simulink library "engine_AMT280_lib"  (Simulink 6.6)
libraries: simulink x5
settings Model: Creator=amurch  LastModifiedBy=amurch

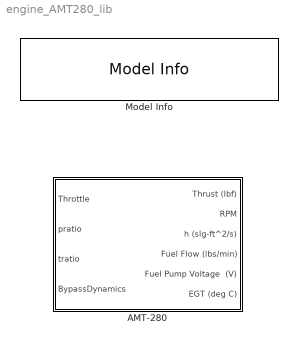
== system engine_AMT280_lib ==
  AMT-280 : Subsystem
      mask init:
      | % Curve fit parameters for AMT-280 Model
      | Coeff_thrust   = [ 5.7372e-05  -5.2629e-03   3.1586e-01  -5.1517e+00];
      | Coeff_throttle = [ -4.3078e-03   1.1110e+00   2.9012e+01];
      | Coeff_fuelflow = [ 1.0140e-04  -1.5867e-03   2.0125e-01];
      | Coeff_tau      = [ -2.2400e-02   2.9948e+00];
      | 
      | 
      | % Equvalent Shaft parameters for engine
      | shaft_dia = 0.75/12.0;       % diameter of rotating turbine in feet 
      | shaft_len = 6.25/12.0;       % length of rotating turbine in feet   
      | density   = 15.2;            % mass density of steel in slugs/ft^3 
      | 
      | fuelpump_table = [ 0.90 1.0 6.4]; %volts, table of fuel pump voltages  - not accurate at the moment 2-4-08
      | fuelflow_table = [0.00 0.1762 1.34044]; %lbs/min,   fuel flow rates corresponding to pump voltages (pumpv_table)
  Model Info : simulink/Model-Wide Utilities/Model Info  SystemSampleTime=-1  InitialBlockCM=None  BlockCM=None  Frame=on  DisplayStringWithTags=|  HorizontalTextAlignment=Center  LeftAlignmentValue=0.5  SourceBlockDiagram=engine_AMT280_lib  TagMaxNumber=20
      | AMT-280 Engine Library
      | 
      | Model Version: %<ModelVersion>
      | Last modifed by %<LastModifiedBy> on %<LastModificationDate>

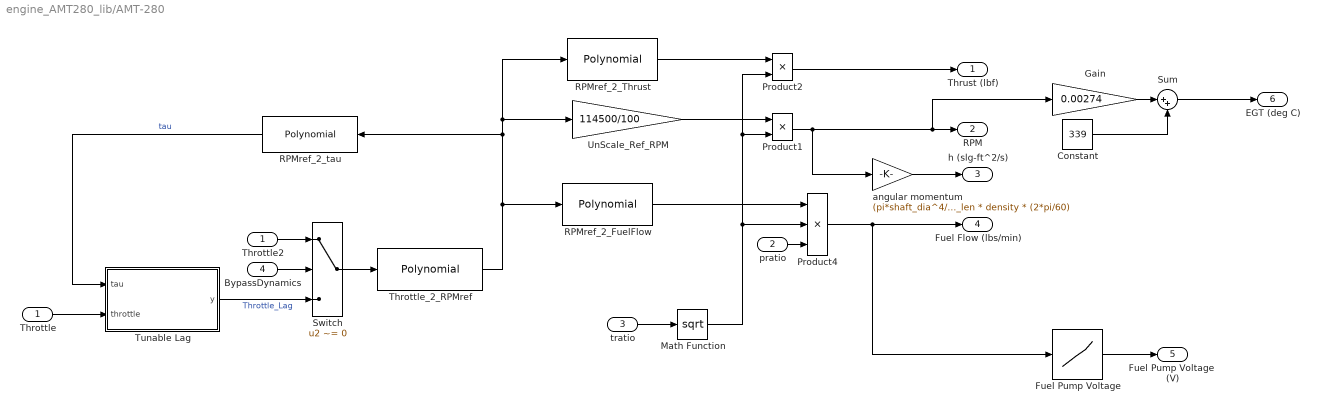
== system engine_AMT280_lib/AMT-280 ==
  Throttle : Inport
  pratio : Inport  Port=2
  tratio : Inport  Port=3
  BypassDynamics : Inport  Port=4
  Constant : Constant  Value=339
  Fuel Pump Voltage : Lookup  InputValues=fuelflow_table  OutputValues=fuelpump_table  LookUpMeth=Interpolation-Use End Values
  Gain : Gain  Gain=0.00274
  Math Function : Math  Operator=sqrt  SaturateOnIntegerOverflow=on
  Product1 : Product  RndMeth=Zero
  Product2 : Product  RndMeth=Zero
  Product4 : Product  Inputs=3  RndMeth=Zero
  RPMref_2_FuelFlow : simulink/Math Operations/Polynomial  coefs=Coeff_fuelflow
  RPMref_2_Thrust : simulink/Math Operations/Polynomial  coefs=Coeff_thrust
  RPMref_2_tau : simulink/Math Operations/Polynomial  Orientation=left  coefs=Coeff_tau
  Sum : Sum  Inputs=|++
  Switch : Switch  Criteria=u2 ~= 0
  Throttle2 : InportShadow  Port=1  LatchByCopyingInsideSignal=off
  Throttle_2_RPMref : simulink/Math Operations/Polynomial  coefs=Coeff_throttle
  Tunable Lag : Subsystem
  UnScale_Ref_RPM : Gain  Gain=114500/100
  angular momentum : Gain  Gain=(pi*shaft_dia^4/32) * shaft_len * density * (2*pi/60)
  Thrust (lbf) : Outport
  RPM : Outport  Port=2
  h (slg-ft^2/s) : Outport  Port=3
  Fuel Flow (lbs/min) : Outport  Port=4
  Fuel Pump Voltage  (V) : Outport  Port=5
  EGT (deg C) : Outport  Port=6
  wires:
  RPMref_2_FuelFlow/1 -> Product4/1
  Product4/1 -> Fuel Flow (lbs/min)/1, Fuel Pump Voltage/1
  Product2/1 -> Thrust (lbf)/1
  Math Function/1 -> Product2/2, Product1/2, Product4/2
  RPMref_2_Thrust/1 -> Product2/1
  tratio/1 -> Math Function/1
  Product1/1 -> angular momentum/1, RPM/1, Gain/1
  pratio/1 -> Product4/3
  UnScale_Ref_RPM/1 -> Product1/1
  angular momentum/1 -> h (slg-ft^2/s)/1
  Throttle_2_RPMref/1 -> RPMref_2_tau/1, UnScale_Ref_RPM/1, RPMref_2_Thrust/1, RPMref_2_FuelFlow/1
  Throttle/1 -> Tunable Lag/2(throttle)
  RPMref_2_tau/1 -> Tunable Lag/1(tau)  "tau"
  Fuel Pump Voltage/1 -> Fuel Pump Voltage  (V)/1
  Sum/1 -> EGT (deg C)/1
  Constant/1 -> Sum/2
  Gain/1 -> Sum/1
  BypassDynamics/1 -> Switch/2
  Throttle2/1 -> Switch/1
  Tunable Lag/1(y) -> Switch/3  "Throttle_Lag"
  Switch/1 -> Throttle_2_RPMref/1

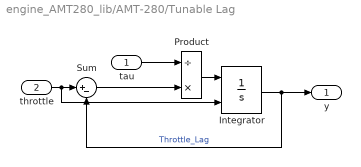
== system engine_AMT280_lib/AMT-280/Tunable Lag ==
  tau : Inport
  throttle : Inport  Port=2
  Integrator : Integrator  InitialConditionSource=external
  Product : Product  Inputs=/*  RndMeth=Zero
  Sum : Sum  Inputs=|+-
  y : Outport
  wires:
  Integrator/1 -> Sum/2, y/1  "Throttle_Lag"
  Product/1 -> Integrator/1
  Sum/1 -> Product/2
  tau/1 -> Product/1
  throttle/1 -> Sum/1, Integrator/2
